simulink model "model"  (R2025a)
settings: Solver=ode4  StartTime=0.0  StopTime=350  FixedStep=fsw.sim.Ts  RelTol=1e-3
values from neighbouring files (symbols this model uses):
  const = load_constants()    [main.m]
  fsw = load_fsw(hw)    [main.m]
  hw = load_hardware()    [main.m]
  ic = load_ic(const, scn)    [main.m]
  scn = load_scenario(const)    [main.m]
  type = scn.type    [main.m]
undefined symbols (not defined in the file or in its folder): FK5, IAU
libraries: vrlib x13, aerolibutil x9, simulink x4, simulink_extras x3, slpidlib x1, aerolibtransform2 x1, aerolibatmos2 x1
settings Model: Creator=procyon  LastModifiedBy=procyon
settings SolverCC: MinimalZcImpactIntegration=on
settings DebuggingCC: ReadBeforeWriteMsg=DisableAll  WriteAfterWriteMsg=DisableAll  WriteAfterReadMsg=DisableAll  MultiTaskDSMMsg=none
settings ModelReferenceCC: UpdateModelReferenceTargets=IfOutOfDate
settings SFSimCC: SFSimEcho=off

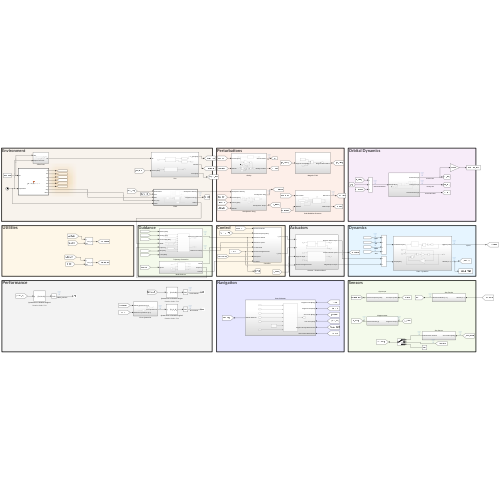
[thumbnail: Simulink's stored preview of the top-level diagram]
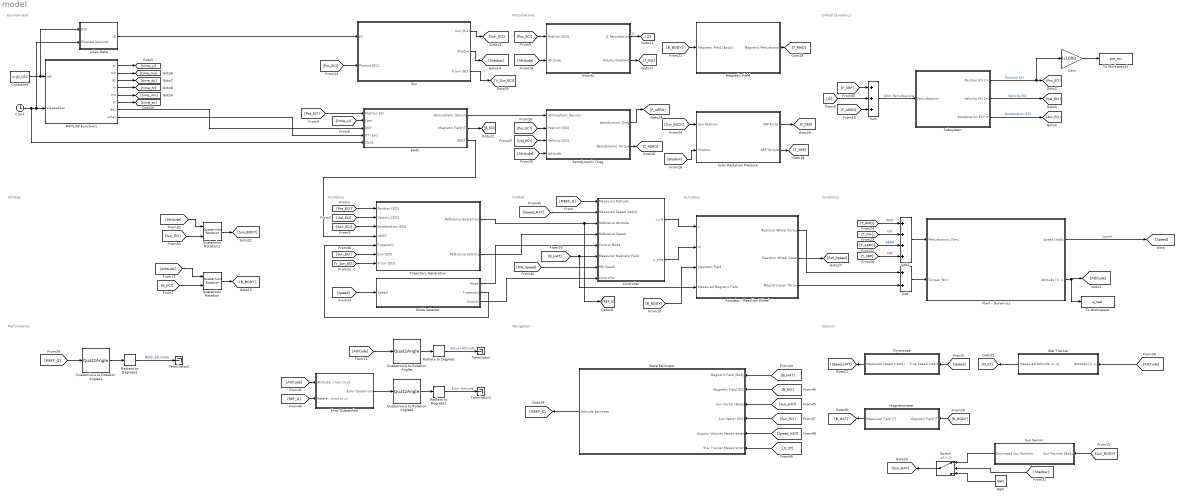
== system model ==
  note: Utilities
  note: Performance
  note: Guidance
  note: Orbital Dynamics
  note: Environment
  note: Navigation
  note: Sensors
  note: Perturbations
  note: Control
  note: Actuators
  note: Dynamics
  Actuator - Reaction Wheel : Subsystem
  Add : Sum
  Add1 : Sum  Inputs=++++
  Aerodynamic Drag : Subsystem
  Clock : Clock
  Constant4 : Constant  Value=ic.JD_UTC
  Controller : Subsystem
  Earth : Subsystem  TreatAsAtomicUnit=on  SystemSampleTime=fsw.sim.Tenv
  Error Quaternion : Subsystem
  Gain : Gain  Gain=1/1000
  Gravity : Subsystem
  Gyroscope : Subsystem
  Julian Date : Subsystem
  MATLAB Function1 : MATLAB Function  TreatAsAtomicUnit=on
  Magnetic Field : Subsystem
  Magnetometer : Subsystem
  Mode Selector : Subsystem
  NaN : Constant  Value=NaN  OutDataTypeStr=Inherit: Inherit via back propagation
  Plant - Dynamics : Subsystem
  Quaternion Rotation : aerolibutil/Quaternion Rotation
  Quaternion Rotation1 : aerolibutil/Quaternion Rotation
  Quaternions to Rotation Angles : Quat2Angle
      settings: AttributesFormatString=Rotation Order: %<rotationOrder>
  Quaternions to Rotation Angles1 : Quat2Angle
      settings: AttributesFormatString=Rotation Order: %<rotationOrder>
  Quaternions to Rotation Angles2 : Quat2Angle
      settings: AttributesFormatString=Rotation Order: %<rotationOrder>
  Radians to Degrees : simulink_extras/Transformations/Radians to Degrees
  Radians to Degrees1 : simulink_extras/Transformations/Radians to Degrees
  Radians to Degrees2 : simulink_extras/Transformations/Radians to Degrees
  Solar Radiation Pressure : Subsystem
  Star Tracker : Subsystem
  State Estimator : Subsystem
  Subsystem : Subsystem
  Sum : Sum  Inputs=+++
  Sun : Subsystem
  Sun Sensor : Subsystem
  Switch : Switch  Criteria=u2 > Threshold  SaturateOnIntegerOverflow=off  InputSameDT=off
  Terminator : Terminator
  Terminator1 : Terminator
  Terminator2 : Terminator
  To Workspace : ToWorkspace  VariableName=q_real  SaveFormat=Timeseries  SampleTime=-1
  To Workspace1 : ToWorkspace  VariableName=pos_eci  SaveFormat=Timeseries  SampleTime=-1
  Trajectory Generation : Subsystem
  wires:
  Plant - Dynamics/1(Speed [rad/s]) -> [Speed]  "Speed"
  Controller/1(u_rw) -> Actuator - Reaction Wheel/1(u)
  Plant - Dynamics/2(Attitude [n. u.]) -> [Attitude], To Workspace/1
  Subsystem/1(Position ECI [m]) -> Gain/1, [Pos_ECI]  "Position ECI"
  Subsystem/3(Acceleration ECI [m]) -> [Acc_ECI]  "Acceleration ECI"
  Subsystem/2(Velocity ECI [m]) -> [Vel_ECI]  "Velocity ECI"
  MATLAB Function1/1(yr) -> [time_yr]
  MATLAB Function1/2(mo) -> [time_mo]
  MATLAB Function1/3(dy) -> [time_dy]
  MATLAB Function1/4(hr) -> [time_hr]
  MATLAB Function1/5(mn) -> [time_mn]
  MATLAB Function1/6(sc) -> [time_sc]
  Constant4/1 -> Julian Date/1(JD0), MATLAB Function1/1(jd0)
  Clock/1 -> Earth/5(Clock), Julian Date/2(Elapsed Seconds), MATLAB Function1/2(elapsedSec)
  [Pos_ECI] -> Trajectory Generation/1(Position [ECI])
  [Vel_ECI] -> Trajectory Generation/2(Velocity [ECI])
  [Acc_ECI] -> Trajectory Generation/3(Acceleration [ECI])
  Trajectory Generation/1(Reference Quaternion) -> [REF_Q], Controller/3(Reference Attitude)
  Trajectory Generation/2(Reference Velocity) -> Controller/4(Reference Speed)
  Gain/1 -> To Workspace1/1
  [Pos_ECI] -> Earth/1(Position ECI)
  [Speed] -> Gyroscope/1(True Speed [rad/s])
  MATLAB Function1/7(doy) -> Earth/3(DOY)
  [time_yr] -> Earth/2(Year)
  MATLAB Function1/8(utSec) -> Earth/4(UT (sec))
  Gravity/1(J2 Perturbation) -> [J2]  "J2"
  [Pos_ECI] -> Gravity/1(Position [ECI])
  Controller/2(u_mtq) -> Actuator - Reaction Wheel/2(m)
  [B_BODY] -> Actuator - Reaction Wheel/3(Magnetic Field)
  Radians to Degrees/1 -> Terminator/1  "Actual Attitude"
  Quaternions to Rotation Angles/1 -> Radians to Degrees/1
  [Attitude] -> Quaternions to Rotation Angles/1
  Actuator - Reaction Wheel/1(Reaction Wheel Torque) -> Add/1
  Actuator - Reaction Wheel/3(Magnetorquer Torque) -> Add/2
  [Speed] -> Mode Selector/1(Speed)
  [Pos_ECI] -> Sun/2(Postion [ECI])
  Julian Date/1(JD) -> Sun/1(JD)
  Sun/1(Sun [ECI]) -> [Sun_ECI]
  Earth/1(Atmospheric Density) -> Aerodynamic Drag/1(Atmospheric Density)
  Sun/2(Shadow) -> [Shadow]
  [Sun_BODY] -> Solar Radiation Pressure/1(Sun Position)
  [Shadow] -> Solar Radiation Pressure/2(Shadow)
  [Attitude] -> Gravity/2(Attitude)
  Earth/3(GMST) -> Trajectory Generation/4(GMST)
  Earth/2(Magnetic Field [T]) -> [B_ECI]
  [B_ECI] -> Quaternion Rotation/2
  [Attitude] -> Quaternion Rotation/1
  Quaternion Rotation/1 -> [B_BODY]
  [B_BODY] -> Magnetic Field/1(Magnetic Field [Body])
  Add/1 -> Plant - Dynamics/2(Torque [Nm])
  Gravity/2(Gravity Gradient) -> [T_GG]
  Solar Radiation Pressure/2(SRP Torque) -> [T_SRP]
  Magnetic Field/1(Magnetic Perturbation) -> [T_RMD]
  [T_SRP] -> Add1/4  "SRP"
  [T_AERO] -> Add1/3  "AERO"
  [T_GG] -> Add1/2  "GG"
  [T_RMD] -> Add1/1  "RMD"
  [Attitude] -> Aerodynamic Drag/4(Attitude)
  [Pos_ECI] -> Aerodynamic Drag/2(Position [ECI])
  [Vel_ECI] -> Aerodynamic Drag/3(Velocity [ECI])
  Add1/1 -> Plant - Dynamics/1(Perturbations [Nm])
  [B_BODY] -> Magnetometer/1(Magnetic Field [T])
  Magnetometer/1(Measured Field [T]) -> [B_HAT]
  [B_HAT] -> Actuator - Reaction Wheel/4(Measured Magnetic Field), Controller/6(Measured Magnetic Field)
  Gyroscope/1(Measured Speed [rad/s]) -> [Speed_HAT]
  [Speed_HAT] -> Controller/2(Measured Speed [rad/s])
  [Shadow] -> Switch/2
  [Attitude] -> Quaternion Rotation1/1
  [Sun_ECI] -> Quaternion Rotation1/2
  Quaternion Rotation1/1 -> [Sun_BODY]
  [Sun_BODY] -> Sun Sensor/1(Sun Position [Body])
  [Attitude] -> Star Tracker/1(Attitude [n. u.])
  Star Tracker/1(Measured Attitude [n. u]) -> [Q_ST]
  Quaternions to Rotation Angles1/1 -> Radians to Degrees1/1
  Radians to Degrees1/1 -> Terminator2/1  "MEKF_Estimate"
  State Estimator/1(Attitude Estimate) -> [MEKF_Q]
  [B_HAT] -> State Estimator/1(Magnetic Field [Body])
  [B_ECI] -> State Estimator/2(Magnetic Field [ECI])
  [Sun_HAT] -> State Estimator/3(Sun Vector [Body])
  [Sun_ECI] -> State Estimator/4(Sun Vector [ECI])
  [Speed_HAT] -> State Estimator/5(Angular Velocity Measurement)
  [Q_ST] -> State Estimator/6(Star Tracker Measurement)
  [MEKF_Q] -> Quaternions to Rotation Angles1/1
  [MEKF_Q] -> Controller/1(Measured Attitude)
  Quaternions to Rotation Angles2/1 -> Radians to Degrees2/1
  Radians to Degrees2/1 -> Terminator1/1  "Error Attitude"
  [REF_Q] -> Error Quaternion/2(Reference Quaternion [n.u])
  [Attitude] -> Error Quaternion/1(Attitude Quaternion [n.u])
  Error Quaternion/1(Error Quaternion) -> Quaternions to Rotation Angles2/1
  Sun Sensor/1(Estimated Sun Position) -> Switch/1
  Switch/1 -> [Sun_HAT]
  NaN/1 -> Switch/3
  Actuator - Reaction Wheel/2(Reaction Wheel Speed) -> [RW_Speed]
  [RW_Speed] -> Controller/7(RW Speed)
  Aerodynamic Drag/2(Aerodynamic Torque) -> [T_AERO]
  Aerodynamic Drag/1(Aerodynamic Drag) -> [F_AERO]
  Solar Radiation Pressure/1(SRP Force) -> [F_SRP]
  Sum/1 -> Subsystem/1(Perturbations)  "Orbit Perturbations"
  [J2] -> Sum/2
  [F_SRP] -> Sum/1
  [F_AERO] -> Sum/3
  Mode Selector/2(Trajectory) -> Trajectory Generation/5(Trajectory)
  Mode Selector/1(Mode) -> Controller/5(Control Mode)
  Mode Selector/3(Control) -> Controller/8(Controller)
  Sun/3(V Sun [ECI]) -> [V_Sun_ECI]
  [V_Sun_ECI] -> Trajectory Generation/7(V Sun [ECI])
  [Sun_ECI] -> Trajectory Generation/6(Sun [ECI])

== system model/Actuator - Reaction Wheel ==
  u : Inport
  m : Inport  Port=2
  Magnetic Field : Inport  Port=3
  Measured Magnetic Field : Inport  Port=4
  DC Motor : Subsystem
  Magnetorquer : Subsystem
  PI Control : Subsystem
  Reaction Wheel Torque : Outport
  Reaction Wheel Speed : Outport  Port=2
  Magnetorquer Torque : Outport  Port=3
  wires:
  DC Motor/2(Speed [rad/s]) -> Reaction Wheel Speed/1, PI Control/2(Motor Speed)
  u/1 -> PI Control/1(Motor Reference)
  Magnetorquer/1(Torque [N.m]) -> Magnetorquer Torque/1
  Magnetic Field/1 -> Magnetorquer/2(Magnetic Field)
  m/1 -> Magnetorquer/1(u_mtq)
  DC Motor/1(Torque [N.m]) -> Reaction Wheel Torque/1
  Measured Magnetic Field/1 -> Magnetorquer/3(Measured Magnetic Field)
  PI Control/1(Voltage) -> DC Motor/1(Voltage)

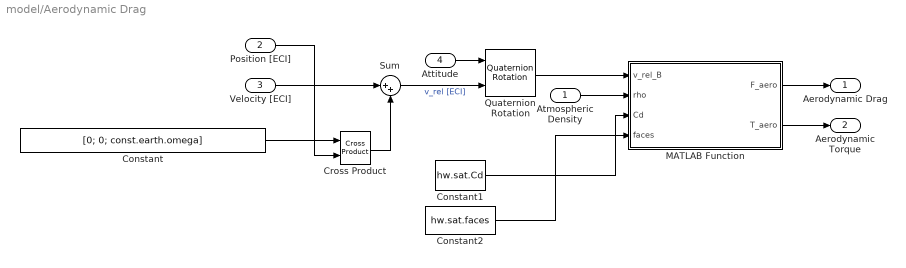
== system model/Aerodynamic Drag ==
  Atmospheric Density : Inport
  Position [ECI] : Inport  Port=2
  Velocity [ECI] : Inport  Port=3
  Attitude : Inport  Port=4
  Constant : Constant  Value=[0; 0; const.earth.omega]
  Constant1 : Constant  Value=hw.sat.Cd
  Constant2 : Constant  Value=hw.sat.faces
  Cross Product : vrlib/Utilities/Cross Product
  MATLAB Function : MATLAB Function  TreatAsAtomicUnit=on
  Quaternion Rotation : aerolibutil/Quaternion Rotation
  Sum : Sum  Inputs=|++
  Aerodynamic Drag : Outport
  Aerodynamic Torque : Outport  Port=2
  wires:
  Constant/1 -> Cross Product/1
  Position [ECI]/1 -> Cross Product/2
  Velocity [ECI]/1 -> Sum/1
  Cross Product/1 -> Sum/2
  Attitude/1 -> Quaternion Rotation/1
  Sum/1 -> Quaternion Rotation/2  "v_rel [ECI]"
  Quaternion Rotation/1 -> MATLAB Function/1(v_rel_B)
  Atmospheric Density/1 -> MATLAB Function/2(rho)
  Constant1/1 -> MATLAB Function/3(Cd)
  Constant2/1 -> MATLAB Function/4(faces)
  MATLAB Function/1(F_aero) -> Aerodynamic Drag/1
  MATLAB Function/2(T_aero) -> Aerodynamic Torque/1

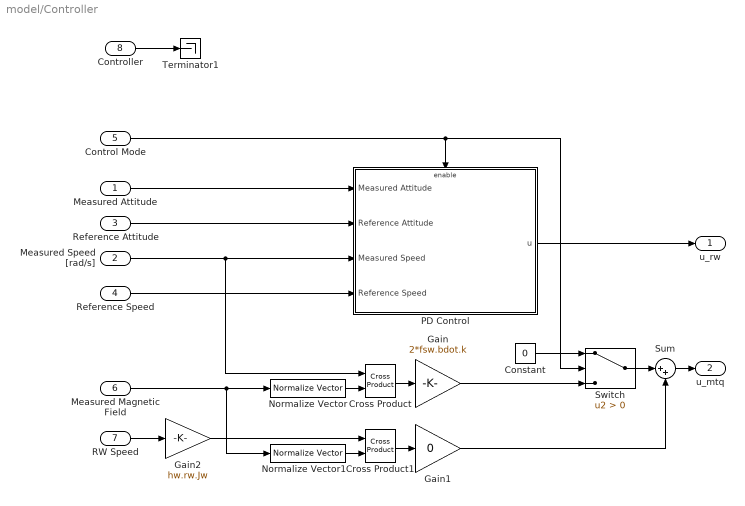
== system model/Controller ==
  Measured Attitude : Inport
  Measured Speed [rad/s] : Inport  Port=2
  Reference Attitude : Inport  Port=3
  Reference Speed : Inport  Port=4
  Control Mode : Inport  Port=5
  Measured Magnetic Field : Inport  Port=6
  RW Speed : Inport  Port=7
  Controller : Inport  Port=8
  Constant : Constant  Value=0
  Cross Product : vrlib/Utilities/Cross Product
  Cross Product1 : vrlib/Utilities/Cross Product
  Gain : Gain  Gain=2*fsw.bdot.k
  Gain1 : Gain  Gain=0
  Gain2 : Gain  Gain=hw.rw.Jw
  Normalize Vector : vrlib/Utilities/Normalize Vector  maxzero=0
  Normalize Vector1 : vrlib/Utilities/Normalize Vector  maxzero=0
  PD Control : Subsystem
  Sum : Sum  Inputs=|++
  Switch : Switch  Criteria=u2 > Threshold  SaturateOnIntegerOverflow=off  InputSameDT=off
  Terminator1 : Terminator
  u_rw : Outport
  u_mtq : Outport  Port=2
  wires:
  Normalize Vector/1 -> Cross Product/2
  Cross Product/1 -> Gain/1
  Measured Magnetic Field/1 -> Normalize Vector1/1, Normalize Vector/1
  RW Speed/1 -> Gain2/1
  Controller/1 -> Terminator1/1
  Measured Attitude/1 -> PD Control/1(Measured Attitude)
  Measured Speed [rad/s]/1 -> PD Control/3(Measured Speed), Cross Product/1
  Reference Attitude/1 -> PD Control/2(Reference Attitude)
  Reference Speed/1 -> PD Control/4(Reference Speed)
  Control Mode/1 -> Switch/2, PD Control/Enable
  Cross Product1/1 -> Gain1/1
  Normalize Vector1/1 -> Cross Product1/2
  Gain2/1 -> Cross Product1/1
  Gain/1 -> Switch/3
  Gain1/1 -> Sum/2
  Switch/1 -> Sum/1
  Sum/1 -> u_mtq/1
  PD Control/1(u) -> u_rw/1
  Constant/1 -> Switch/1

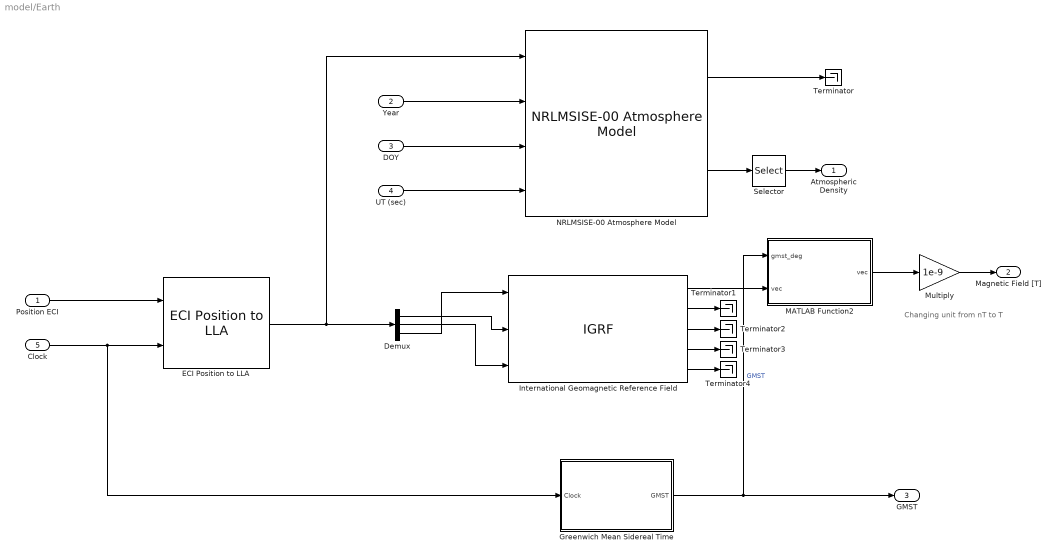
== system model/Earth ==
  note: Changing unit from nT to T
  Position ECI : Inport
  Year : Inport  Port=2
  DOY : Inport  Port=3
  UT (sec) : Inport  Port=4
  Clock : Inport  Port=5
  Demux : Demux  Outputs=3
  ECI Position to LLA : aerolibtransform2/ECI Position to LLA  red=IAU-76/FK5  year=2000  month=January  day=1  hour=12  min=0  sec=0  deltaT=Sec  errorflag=Error  extraparamflag=off  eunits=Metric (MKS)  earthmodel=WGS84  flat=1/298.257223563  eqradius=6378137
      settings: AttributesFormatString=%<red>
  Greenwich Mean Sidereal Time : Subsystem
  International Geomagnetic Reference Field : IGRF  time_in=off  month=January  day=1  year=2000  sv_out=off
      settings: AttributesFormatString=%<generation>
  MATLAB Function2 : MATLAB Function  TreatAsAtomicUnit=on
  Multiply : Gain  Gain=1e-9
  NRLMSISE-00 Atmosphere Model : aerolibatmos2/NRLMSISE-00 Atmosphere Model  units=Metric (MKS)  lst_input=off  flux_ap_input=off  flags_input=Internal  flags=ones(1,23)  oxygen_in=off  action=Warning
  Selector : Selector  InputPortWidth=9  IndexOptions=Index vector (dialog)  Indices=[6]  OutputSizes=1
  Terminator{,1..4} (5 alike) : Terminator
  Atmospheric Density : Outport
  Magnetic Field [T] : Outport  Port=2
  GMST : Outport  Port=3
  wires:
  ECI Position to LLA/1 -> Demux/1, NRLMSISE-00 Atmosphere Model/1
  NRLMSISE-00 Atmosphere Model/1 -> Terminator/1
  Position ECI/1 -> ECI Position to LLA/1
  Clock/1 -> Greenwich Mean Sidereal Time/1(Clock), ECI Position to LLA/2
  UT (sec)/1 -> NRLMSISE-00 Atmosphere Model/4
  DOY/1 -> NRLMSISE-00 Atmosphere Model/3
  Year/1 -> NRLMSISE-00 Atmosphere Model/2
  Demux/3 -> International Geomagnetic Reference Field/1
  Demux/1 -> International Geomagnetic Reference Field/2
  Demux/2 -> International Geomagnetic Reference Field/3
  International Geomagnetic Reference Field/2 -> Terminator1/1
  International Geomagnetic Reference Field/3 -> Terminator2/1
  International Geomagnetic Reference Field/4 -> Terminator3/1
  International Geomagnetic Reference Field/5 -> Terminator4/1
  NRLMSISE-00 Atmosphere Model/2 -> Selector/1
  Selector/1 -> Atmospheric Density/1
  MATLAB Function2/1(vec) -> Multiply/1
  Greenwich Mean Sidereal Time/1(GMST) -> MATLAB Function2/1(gmst_deg), GMST/1  "GMST"
  International Geomagnetic Reference Field/1 -> MATLAB Function2/2("vec ")
  Multiply/1 -> Magnetic Field [T]/1

== system model/Error Quaternion ==
  Attitude Quaternion [n.u] : Inport
  Reference Quaternion [n.u] : Inport  Port=2
  Quaternion Inverse : aerolibutil/Quaternion Inverse
  Quaternion Multiplication : aerolibutil/Quaternion Multiplication
  Error Quaternion : Outport
  wires:
  Reference Quaternion [n.u]/1 -> Quaternion Inverse/1
  Quaternion Multiplication/1 -> Error Quaternion/1
  Quaternion Inverse/1 -> Quaternion Multiplication/2
  Attitude Quaternion [n.u]/1 -> Quaternion Multiplication/1

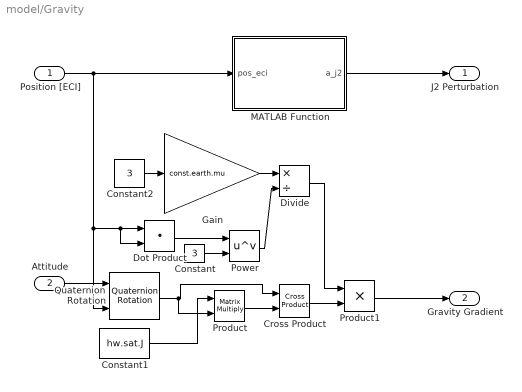
== system model/Gravity ==
  Position [ECI] : Inport
  Attitude : Inport  Port=2
  Constant : Constant  Value=3
  Constant1 : Constant  Value=hw.sat.J
  Constant2 : Constant  Value=3
  Cross Product : vrlib/Utilities/Cross Product
  Divide : Product  Inputs=*/
  Dot Product : DotProduct  OutDataTypeStr=Inherit: Inherit via internal rule
  Gain : Gain  Gain=const.earth.mu
  MATLAB Function : MATLAB Function  TreatAsAtomicUnit=on
  Power : Math  Operator=pow
  Product : Product  Multiplication=Matrix(*)
  Product1 : Product
  Quaternion Rotation : aerolibutil/Quaternion Rotation
  J2 Perturbation : Outport
  Gravity Gradient : Outport  Port=2
  wires:
  MATLAB Function/1(a_j2) -> J2 Perturbation/1
  Attitude/1 -> Quaternion Rotation/1
  Position [ECI]/1 -> MATLAB Function/1(pos_eci), Quaternion Rotation/2, Dot Product/2, Dot Product/1
  Power/1 -> Divide/2
  Dot Product/1 -> Power/1
  Constant/1 -> Power/2
  Quaternion Rotation/1 -> Product/2, Cross Product/1
  Constant1/1 -> Product/1
  Product/1 -> Cross Product/2
  Cross Product/1 -> Product1/2
  Constant2/1 -> Gain/1
  Gain/1 -> Divide/1
  Divide/1 -> Product1/1
  Product1/1 -> Gravity Gradient/1

== system model/Gyroscope ==
  True Speed [rad/s] : Inport
  Add : Sum  Inputs=+++
  Bias : simulink/Sources/Band-Limited White Noise  Cov=hw.gyro.sigma_bias^2  Ts=fsw.sim.Ts  seed=[23341]
  Integrator : Integrator  InitialCondition=hw.gyro.bias0
  Noise : simulink/Sources/Band-Limited White Noise  Cov=hw.gyro.sigma_noise^2  Ts=fsw.sim.Ts  seed=[23341]
  Measured Speed [rad/s] : Outport
  wires:
  True Speed [rad/s]/1 -> Add/2
  Add/1 -> Measured Speed [rad/s]/1
  Noise/1 -> Add/1
  Integrator/1 -> Add/3
  Bias/1 -> Integrator/1

== system model/Julian Date ==
  JD0 : Inport
  Elapsed Seconds : Inport  Port=2
  Constant : Constant  Value=86400
  Divide : Product  Inputs=*/
  Sum : Sum  Inputs=|++
  JD : Outport
  wires:
  Elapsed Seconds/1 -> Divide/1
  Constant/1 -> Divide/2
  JD0/1 -> Sum/1
  Sum/1 -> JD/1
  Divide/1 -> Sum/2

== system model/Magnetic Field ==
  Magnetic Field [Body] : Inport
  Constant : Constant  Value=hw.sat.rmd
  Cross Product : vrlib/Utilities/Cross Product
  Magnetic Perturbation : Outport
  wires:
  Cross Product/1 -> Magnetic Perturbation/1
  Magnetic Field [Body]/1 -> Cross Product/2
  Constant/1 -> Cross Product/1

== system model/Magnetometer ==
  Magnetic Field [T] : Inport
  Add : Sum  Inputs=+++
  Constant : Constant  Value=hw.mag.bias
  Noise : simulink/Sources/Band-Limited White Noise  Cov=hw.mag.sigma_noise^2 * hw.mag.dt  Ts=fsw.sim.Ts  seed=[23341]
  Zero-Order Hold : ZeroOrderHold  SampleTime=hw.mag.dt
  Measured Field [T] : Outport
  wires:
  Add/1 -> Zero-Order Hold/1
  Noise/1 -> Add/1
  Constant/1 -> Add/3
  Magnetic Field [T]/1 -> Add/2
  Zero-Order Hold/1 -> Measured Field [T]/1

== system model/Mode Selector ==
  Speed : Inport
  Clock : Clock
  Constant : Constant  Value=type
  MATLAB Function : MATLAB Function  TreatAsAtomicUnit=on
  Mode : Outport
  Trajectory : Outport  Port=2
  Control : Outport  Port=3
  wires:
  Speed/1 -> MATLAB Function/1(w)
  MATLAB Function/1(mode) -> Mode/1
  MATLAB Function/3(ctrl_select) -> Control/1
  MATLAB Function/2(traj_select) -> Trajectory/1
  Constant/1 -> MATLAB Function/2(scn_type)
  Clock/1 -> MATLAB Function/3(t)

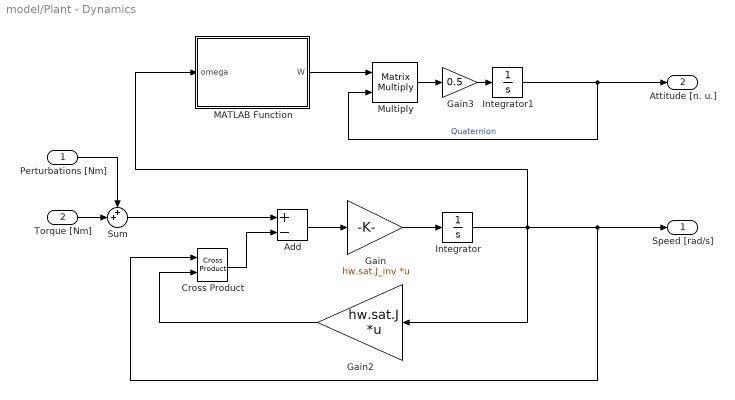
== system model/Plant - Dynamics ==
  Perturbations [Nm] : Inport
  Torque [Nm] : Inport  Port=2
  Add : Sum  Inputs=+-
  Cross Product : vrlib/Utilities/Cross Product
  Gain : Gain  Gain=hw.sat.J_inv  Multiplication=Matrix(K*u) (u vector)
  Gain2 : Gain  Gain=hw.sat.J  Multiplication=Matrix(K*u) (u vector)
  Gain3 : Gain  Gain=0.5
  Integrator : Integrator  InitialCondition=ic.w0
  Integrator1 : Integrator  InitialCondition=ic.q0
  MATLAB Function : MATLAB Function  TreatAsAtomicUnit=on
  Multiply : Product  Inputs=**  Multiplication=Matrix(*)
  Sum : Sum  Inputs=++|
  Speed [rad/s] : Outport
  Attitude [n. u.] : Outport  Port=2
  wires:
  Add/1 -> Gain/1
  Cross Product/1 -> Add/2
  Gain2/1 -> Cross Product/2
  Integrator/1 -> MATLAB Function/1(omega), Cross Product/1, Speed [rad/s]/1, Gain2/1
  MATLAB Function/1(W) -> Multiply/1
  Multiply/1 -> Gain3/1
  Integrator1/1 -> Attitude [n. u.]/1, Multiply/2  "Quaternion"
  Gain3/1 -> Integrator1/1
  Gain/1 -> Integrator/1
  Perturbations [Nm]/1 -> Sum/1
  Torque [Nm]/1 -> Sum/2
  Sum/1 -> Add/1

== system model/Solar Radiation Pressure ==
  Sun Position : Inport
  Shadow : Inport  Port=2
  Constant : Constant  Value=const.phys.c
  Constant1 : Constant  Value=const.sun.solar_const
  Constant2 : Constant  Value=hw.sat.faces
  MATLAB Function : MATLAB Function  TreatAsAtomicUnit=on
  SRP Force : Outport
  SRP Torque : Outport  Port=2
  wires:
  Constant/1 -> MATLAB Function/3(c)
  Constant1/1 -> MATLAB Function/2(solar_const)
  Constant2/1 -> MATLAB Function/4(faces)
  Sun Position/1 -> MATLAB Function/1(s_B)
  MATLAB Function/2(T_srp) -> SRP Torque/1
  MATLAB Function/1(F_srp) -> SRP Force/1

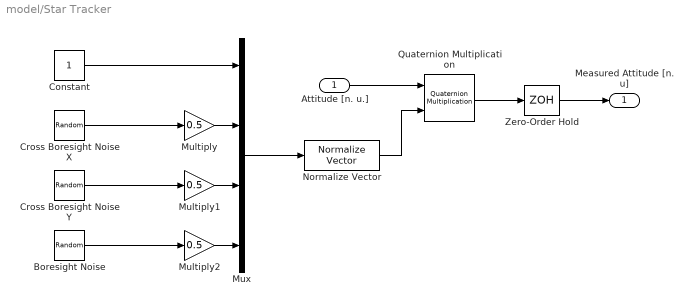
== system model/Star Tracker ==
  Attitude [n. u.] : Inport
  Boresight Noise : RandomNumber  Variance=hw.st.sigma_bore^2  SampleTime=hw.st.dt
  Constant : Constant
  Cross Boresight Noise X : RandomNumber  Variance=hw.st.sigma_cross^2  SampleTime=hw.st.dt
  Cross Boresight Noise Y : RandomNumber  Variance=hw.st.sigma_cross^2  SampleTime=hw.st.dt
  Multiply : Gain  Gain=0.5
  Multiply1 : Gain  Gain=0.5
  Multiply2 : Gain  Gain=0.5
  Mux : Mux
  Normalize Vector : vrlib/Utilities/Normalize Vector  maxzero=0
  Quaternion Multiplication : aerolibutil/Quaternion Multiplication
  Zero-Order Hold : ZeroOrderHold  SampleTime=0.1
  Measured Attitude [n. u] : Outport
  wires:
  Constant/1 -> Mux/1
  Cross Boresight Noise X/1 -> Multiply/1
  Cross Boresight Noise Y/1 -> Multiply1/1
  Boresight Noise/1 -> Multiply2/1
  Mux/1 -> Normalize Vector/1
  Attitude [n. u.]/1 -> Quaternion Multiplication/1
  Multiply/1 -> Mux/2
  Multiply1/1 -> Mux/3
  Multiply2/1 -> Mux/4
  Quaternion Multiplication/1 -> Zero-Order Hold/1
  Normalize Vector/1 -> Quaternion Multiplication/2
  Zero-Order Hold/1 -> Measured Attitude [n. u]/1

== system model/State Estimator ==
  Magnetic Field [Body] : Inport
  Magnetic Field [ECI] : Inport  Port=2
  Sun Vector [Body] : Inport  Port=3
  Sun Vector [ECI] : Inport  Port=4
  Angular Velocity Measurement : Inport  Port=5
  Star Tracker Measurement : Inport  Port=6
  Constant : Constant  Value=fsw.sim.Ts
  MATLAB Function : MATLAB Function  TreatAsAtomicUnit=on
  Attitude Estimate : Outport
  wires:
  Magnetic Field [Body]/1 -> MATLAB Function/1(mag_b)
  Magnetic Field [ECI]/1 -> MATLAB Function/2(mag_ref)
  Sun Vector [Body]/1 -> MATLAB Function/3(sun_b)
  Sun Vector [ECI]/1 -> MATLAB Function/4(sun_ref)
  Angular Velocity Measurement/1 -> MATLAB Function/5(gyro)
  Constant/1 -> MATLAB Function/6(dt)
  Star Tracker Measurement/1 -> MATLAB Function/7(q_st)
  MATLAB Function/1(q_est) -> Attitude Estimate/1

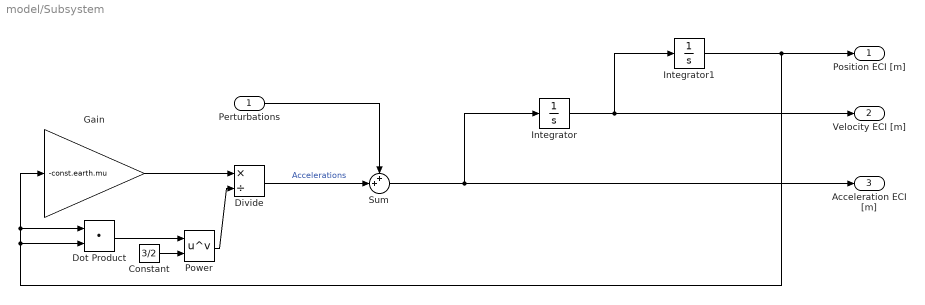
== system model/Subsystem ==
  Perturbations : Inport
  Constant : Constant  Value=3/2
  Divide : Product  Inputs=*/
  Dot Product : DotProduct  OutDataTypeStr=Inherit: Inherit via internal rule
  Gain : Gain  Gain=-const.earth.mu
  Integrator : Integrator  InitialCondition=ic.v0_I
  Integrator1 : Integrator  InitialCondition=ic.r0_I
  Power : Math  Operator=pow
  Sum : Sum  Inputs=++|
  Position ECI [m] : Outport
  Velocity ECI [m] : Outport  Port=2
  Acceleration ECI [m] : Outport  Port=3
  wires:
  Integrator/1 -> Integrator1/1, Velocity ECI [m]/1
  Integrator1/1 -> Dot Product/2, Dot Product/1, Gain/1, Position ECI [m]/1
  Dot Product/1 -> Power/1
  Gain/1 -> Divide/1
  Constant/1 -> Power/2
  Power/1 -> Divide/2
  Perturbations/1 -> Sum/1
  Divide/1 -> Sum/2  "Accelerations"
  Sum/1 -> Acceleration ECI [m]/1, Integrator/1

== system model/Sun ==
  JD : Inport
  Postion [ECI] : Inport  Port=2
  Eclipse Shadow Model (Cylindrical) : EclipseShadowModel  shadowModel=Cylindrical
  Normalize Vector : vrlib/Utilities/Normalize Vector  maxzero=0
  Normalize Vector1 : vrlib/Utilities/Normalize Vector  maxzero=0
  Planetary Ephemeris : PlanetaryEphem  target=Sun
  Sun [ECI] : Outport
  Shadow : Outport  Port=2
  V Sun [ECI] : Outport  Port=3
  wires:
  Planetary Ephemeris/1 -> Normalize Vector/1
  JD/1 -> Planetary Ephemeris/1
  Planetary Ephemeris/2 -> Normalize Vector1/1
  Postion [ECI]/1 -> Eclipse Shadow Model (Cylindrical)/1
  Eclipse Shadow Model (Cylindrical)/1 -> Shadow/1
  Normalize Vector/1 -> Sun [ECI]/1
  Normalize Vector1/1 -> V Sun [ECI]/1

== system model/Sun Sensor ==
  Sun Position [Body] : Inport
  Add : Sum
  Noise : simulink/Sources/Band-Limited White Noise  Cov=hw.ss.sigma_angle^2  Ts=fsw.sim.Ts  seed=[23341]
  Normalize Vector : vrlib/Utilities/Normalize Vector  maxzero=0
  Zero-Order Hold : ZeroOrderHold  SampleTime=hw.ss.dt
  Estimated Sun Position : Outport
  wires:
  Sun Position [Body]/1 -> Add/2
  Noise/1 -> Add/1
  Add/1 -> Normalize Vector/1
  Normalize Vector/1 -> Zero-Order Hold/1
  Zero-Order Hold/1 -> Estimated Sun Position/1

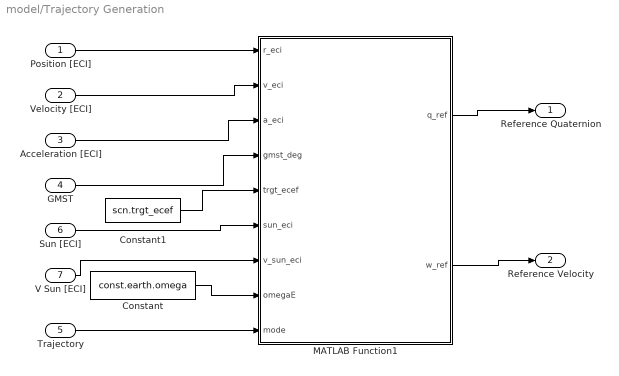
== system model/Trajectory Generation ==
  Position [ECI] : Inport
  Velocity [ECI] : Inport  Port=2
  Acceleration [ECI] : Inport  Port=3
  GMST : Inport  Port=4
  Trajectory : Inport  Port=5
  Sun [ECI] : Inport  Port=6
  V Sun [ECI] : Inport  Port=7
  Constant : Constant  Value=const.earth.omega
  Constant1 : Constant  Value=scn.trgt_ecef
  MATLAB Function1 : MATLAB Function  TreatAsAtomicUnit=on
  Reference Quaternion : Outport
  Reference Velocity : Outport  Port=2
  wires:
  Position [ECI]/1 -> MATLAB Function1/1(r_eci)
  Velocity [ECI]/1 -> MATLAB Function1/2(v_eci)
  Acceleration [ECI]/1 -> MATLAB Function1/3(a_eci)
  GMST/1 -> MATLAB Function1/4(gmst_deg)
  Constant1/1 -> MATLAB Function1/5(trgt_ecef)
  Constant/1 -> MATLAB Function1/8(omegaE)
  MATLAB Function1/1(q_ref) -> Reference Quaternion/1
  MATLAB Function1/2(w_ref) -> Reference Velocity/1
  Trajectory/1 -> MATLAB Function1/9(mode)
  Sun [ECI]/1 -> MATLAB Function1/6(sun_eci)
  V Sun [ECI]/1 -> MATLAB Function1/7(v_sun_eci)

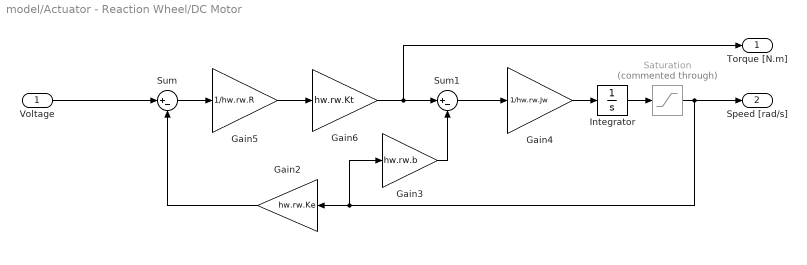
== system model/Actuator - Reaction Wheel/DC Motor ==
  Voltage : Inport
  Gain2 : Gain  Gain=hw.rw.Ke
  Gain3 : Gain  Gain=hw.rw.b
  Gain4 : Gain  Gain=1/hw.rw.Jw
  Gain5 : Gain  Gain=1/hw.rw.R
  Gain6 : Gain  Gain=hw.rw.Kt
  Integrator : Integrator
  Saturation : Saturate  Commented=through  UpperLimit=1000  LowerLimit=-1000
  Sum : Sum  Inputs=|+-
  Sum1 : Sum  Inputs=|+-
  Torque [N.m] : Outport
  Speed [rad/s] : Outport  Port=2
  wires:
  Voltage/1 -> Sum/1
  Gain2/1 -> Sum/2
  Sum/1 -> Gain5/1
  Gain6/1 -> Torque [N.m]/1, Sum1/1
  Integrator/1 -> Saturation/1
  Gain4/1 -> Integrator/1
  Gain5/1 -> Gain6/1
  Sum1/1 -> Gain4/1
  Gain3/1 -> Sum1/2
  Saturation/1 -> Gain3/1, Gain2/1, Speed [rad/s]/1

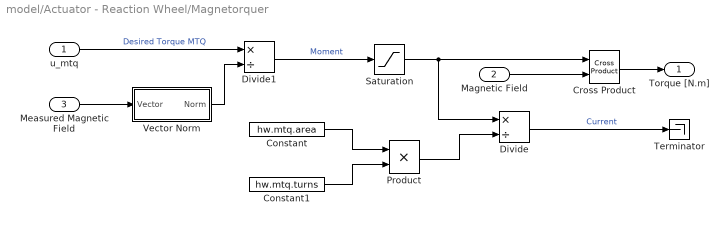
== system model/Actuator - Reaction Wheel/Magnetorquer ==
  u_mtq : Inport
  Magnetic Field : Inport  Port=2
  Measured Magnetic Field : Inport  Port=3
  Constant : Constant  Value=hw.mtq.area
  Constant1 : Constant  Value=hw.mtq.turns
  Cross Product : vrlib/Utilities/Cross Product
  Divide : Product  Inputs=*/
  Divide1 : Product  Inputs=*/
  Product : Product
  Saturation : Saturate  UpperLimit=hw.mtq.m_max  LowerLimit=-hw.mtq.m_max
  Terminator : Terminator
  Vector Norm : Subsystem
  Torque [N.m] : Outport
  wires:
  Magnetic Field/1 -> Cross Product/2
  Cross Product/1 -> Torque [N.m]/1
  Constant/1 -> Product/1
  Constant1/1 -> Product/2
  Product/1 -> Divide/2
  Divide/1 -> Terminator/1  "Current"
  Saturation/1 -> Cross Product/1, Divide/1
  Vector Norm/1(Norm) -> Divide1/2
  Measured Magnetic Field/1 -> Vector Norm/1(Vector)
  u_mtq/1 -> Divide1/1  "Desired Torque MTQ"
  Divide1/1 -> Saturation/1  "Moment"

== system model/Actuator - Reaction Wheel/PI Control ==
  Motor Reference : Inport
  Motor Speed : Inport  Port=2
  Gain : Gain  Gain=1/hw.rw.Jw
  Integrator : Integrator
  PID Controller : slpidlib/PID Controller  Controller=PI  Form=Parallel  TimeDomain=Continuous-time  UseExternalTs=off  SampleTime=-1  IntegratorMethod=Forward Euler  FilterMethod=Forward Euler  ControllerParametersSource=internal  P=0.3  I=2.3  UseKiTs=off  D=0  UseExternalDerivativeSource=off  N=100  UseFilter=on  TunerSelectOption=Transfer Function Based (PID Tuner App)  InitialConditionSource=internal  InitialConditionForIntegrator=0  InitialConditionForFilter=0  DifferentiatorICPrevScaledInput=0  ExternalReset=none  TrackingMode=off  Kt=1  LimitOutput=off  SatLimitsSource=internal  UpperSaturationLimit=inf  LowerSaturationLimit=-inf  LinearizeAsGain=on  AntiWindupMode=none  Kb=1  LimitIntegrator=off  UpperIntegratorSaturationLimit=inf  LowerIntegratorSaturationLimit=-inf  POutMin=[]  POutMax=[]  IOutMin=[]  IOutMax=[]  DOutMin=[]  DOutMax=[]  NOutMin=[]  NOutMax=[]  SumOutMin=[]  SumOutMax=[]  SaturationOutMin=[]  SaturationOutMax=[]  PParamMin=[]  PParamMax=[]  IParamMin=[]  IParamMax=[]  DParamMin=[]  DParamMax=[]  NParamMin=[]  NParamMax=[]  KbParamMin=[]  KbParamMax=[]  KtParamMin=[]  KtParamMax=[]  KbOutMin=[]  KbOutMax=[]  KtOutMin=[]  KtOutMax=[]  IntegratorOutMin=[]  IntegratorOutMax=[]  FilterOutMin=[]  FilterOutMax=[]  SumI1OutMin=[]  SumI1OutMax=[]  SumI2OutMin=[]  SumI2OutMax=[]  SumI3OutMin=[]  SumI3OutMax=[]  SumI4OutMin=[]  SumI4OutMax=[]  SumDOutMin=[]  SumDOutMax=[]  DifferentiatorOutMin=[]  DifferentiatorOutMax=[]  FilterDiffOutCoefMin=[]  FilterDiffOutCoefMax=[]  ReciprocalOutMin=[]  ReciprocalOutMax=[]  SumDenOutMin=[]  SumDenOutMax=[]  SumNumOutMin=[]  SumNumOutMax=[]  DivideOutMin=[]  DivideOutMax=[]  UdiffTsProdOutMin=[]  UdiffTsProdOutMax=[]  NTsProdOutMin=[]  NTsProdOutMax=[]  UintegralTsProdOutMin=[]  UintegralTsProdOutMax=[]  UngainTsProdOutMin=[]  UngainTsProdOutMax=[]  ClampingZeroOutDataTypeStr=Inherit: Inherit via back propagation  ClampingZeroOutMin=[]  ClampingZeroOutMax=[]  FilterDenConstantOutDataTypeStr=Inherit: Inherit via back propagation  FilterDenConstantOutMin=[]  FilterDenConstantOutMax=[]  PCopyOutDataTypeStr=Inherit: Inherit via back propagation  PCopyOutMin=[]  PCopyOutMax=[]  NCopyOutDataTypeStr=Inherit: Inherit via back propagation  NCopyOutMin=[]  NCopyOutMax=[]  IntegratorContinuousStateAttributes=''  IntegratorStateMustResolveToSignalObject=off  IntegratorRTWStateStorageClass=Auto  FilterContinuousStateAttributes=''  FilterStateMustResolveToSignalObject=off  FilterRTWStateStorageClass=Auto  ParallelPVariant=InternalParameters  IdealPVariant=Disabled  IVariant=InternalParameters  DVariant=Disabled  IntegratorVariant=Continuous  SatVariant=Disabled  AWVariant=Passthrough  PCopyVariant=Disabled  TRVariant=Disabled  FdbkBlocksVariant=Forward  IdealPFdbkVariant=Disabled  SatFdbkVariant=Disabled  DerivativeFilterVariant=Disabled  NVariant=Disabled  NCopyVariant=Disabled_SignalSpec  FilterICVariant=Disabled  IntegratorICVariant=InternalICs  ExternalResetVariant=Disabled  TRSumVariant=Passthrough  SumFdbkVariant=Disabled  SumVariant=Sum_PI  TsampFilterVariant=InternalTs  TsampNgainVariant=Passthrough  TsampIntegralVariant=Disabled_SignalSpec  ExternalSaturationOutDataTypeStr=Inherit: Same as second input  DerivativeSourceVariant=Disabled  PreIntVariant=InternalPreInt
  Sum : Sum  Inputs=|+-
  Voltage : Outport
  wires:
  Motor Reference/1 -> Gain/1
  Gain/1 -> Integrator/1
  Integrator/1 -> Sum/1
  Motor Speed/1 -> Sum/2
  Sum/1 -> PID Controller/1
  PID Controller/1 -> Voltage/1

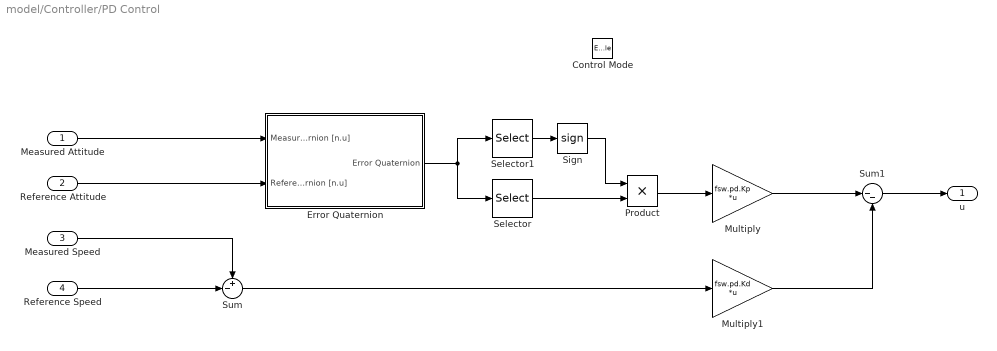
== system model/Controller/PD Control ==
  Measured Attitude : Inport
  Reference Attitude : Inport  Port=2
  Measured Speed : Inport  Port=3
  Reference Speed : Inport  Port=4
  Control Mode : EnablePort
  Error Quaternion : Subsystem
  Multiply : Gain  Gain=fsw.pd.Kp  Multiplication=Matrix(K*u) (u vector)
  Multiply1 : Gain  Gain=fsw.pd.Kd  Multiplication=Matrix(K*u) (u vector)
  Product : Product
  Selector : Selector  InputPortWidth=4  IndexOptions=Index vector (dialog)  Indices=[2 3 4]  OutputSizes=1
  Selector1 : Selector  InputPortWidth=4  IndexOptions=Index vector (dialog)  Indices=[1]  OutputSizes=1
  Sign : Signum
  Sum : Sum  Inputs=+-|
  Sum1 : Sum  Inputs=|--
  u : Outport
  wires:
  Error Quaternion/1(Error Quaternion) -> Selector1/1, Selector/1
  Selector1/1 -> Sign/1
  Selector/1 -> Product/2
  Product/1 -> Multiply/1
  Multiply/1 -> Sum1/1
  Sum/1 -> Multiply1/1
  Sign/1 -> Product/1
  Measured Attitude/1 -> Error Quaternion/1(Measured Quaternion [n.u])
  Reference Attitude/1 -> Error Quaternion/2(Reference Quaternion [n.u])
  Measured Speed/1 -> Sum/1
  Reference Speed/1 -> Sum/2
  Multiply1/1 -> Sum1/2
  Sum1/1 -> u/1

== system model/Earth/Greenwich Mean Sidereal Time ==
  Clock : Inport
  Add : Sum
  Constant : Constant  Value=ic.gmst0_deg
  Constant1 : Constant  Value=const.earth.omega
  Constant2 : Constant  Value=360
  Gain : Gain  Gain=180 / pi
  Mod : Math  Operator=mod
  Product : Product
  GMST : Outport
  wires:
  Clock/1 -> Product/2
  Constant1/1 -> Product/1
  Product/1 -> Gain/1
  Gain/1 -> Add/2
  Constant/1 -> Add/1
  Mod/1 -> GMST/1
  Add/1 -> Mod/1
  Constant2/1 -> Mod/2

== system model/Actuator - Reaction Wheel/Magnetorquer/Vector Norm ==
  Vector : Inport
  Dot Product : DotProduct  OutDataTypeStr=Inherit: Inherit via internal rule
  Square Root : Sqrt
  Norm : Outport
  wires:
  Vector/1 -> Dot Product/2, Dot Product/1
  Dot Product/1 -> Square Root/1
  Square Root/1 -> Norm/1

== system model/Controller/PD Control/Error Quaternion ==
  Measured Quaternion [n.u] : Inport
  Reference Quaternion [n.u] : Inport  Port=2
  Quaternion Inverse : aerolibutil/Quaternion Inverse
  Quaternion Multiplication : aerolibutil/Quaternion Multiplication
  Error Quaternion : Outport
  wires:
  Reference Quaternion [n.u]/1 -> Quaternion Inverse/1
  Quaternion Multiplication/1 -> Error Quaternion/1
  Quaternion Inverse/1 -> Quaternion Multiplication/2
  Measured Quaternion [n.u]/1 -> Quaternion Multiplication/1

== matlab function model/Trajectory Generation/MATLAB Function1 ==
  data: r_eci input; q_ref output; v_eci input; a_eci input; gmst_deg input; trgt_ecef input; sun_eci input; v_sun_eci input; omegaE input; mode input; w_ref output
%#codegen
function [q_ref, w_ref] = trajectory(r_eci, v_eci, a_eci, gmst_deg, trgt_ecef, sun_eci, v_sun_eci, omegaE, mode)

    q_ref = zeros(4,1);
    w_ref = zeros(3,1);

    r_eci = r_eci(:);
    v_eci = v_eci(:);
    a_eci = a_eci(:);
    sun_eci = sun_eci(:);
    v_sun_eci = v_sun_eci(:);

    switch mode
        case 1 % Inertial Pointing mode, satellite goes to origin
            q_ref = [1; 0; 0; 0];
            w_ref = [0; 0; 0];
        case 2 % Nadir Pointing mode, satellite points to Earth
            [q_ref, w_ref] = nadir_pointing(r_eci, v_eci, a_eci);
        case 3 % Sun Pointing mode, satellite points to the Sun
            [q_ref, w_ref] = sun_pointing(sun_eci, v_sun_eci, r_eci, v_eci, a_eci);
        case 4 % Target Tracking mode, satellite points to ground station
            [q_ref, w_ref] = target_tracking(gmst_deg, trgt_ecef, r_eci, v_eci, omegaE);
        otherwise
            q_ref = [1; 0; 0; 0];
            w_ref = [0; 0; 0];
    end

== matlab function model/Aerodynamic Drag/MATLAB Function ==
  data: F_aero output; v_rel_B input; T_aero output; rho input; Cd input; faces input
function [F_aero, T_aero] = aero_drag(v_rel_B, rho, Cd, faces)

    V = norm(v_rel_B);
    if V < eps
        F_aero = zeros(3,1);
        T_aero = zeros(3,1);
        return;
    end

    F_aero = zeros(3,1);
    T_aero = zeros(3,1);
    N = size(faces, 1);

    for k = 1:N
        n_k   = faces(k, 1:3)';
        A_k   = faces(k, 4);
        r_k   = faces(k, 5:7)';

        cos_alpha = dot(v_rel_B, n_k) / V;

        if cos_alpha > 0
            F_k = -0.5 * rho * Cd * A_k * cos_alpha * V * v_rel_B;
            F_aero = F_aero + F_k;
            T_aero = T_aero + cross(r_k, F_k);
        end
    end

end

== matlab function model/Plant - Dynamics/MATLAB Function ==
  data: omega input; W output
function W = omegaMat(omega)
%OMEGAMAT  Quaternion kinematic matrix (scalar-first convention)
%
%   Using the definition:
%       W(ω) = [  0      -ωᵀ
%                 ω   [ω×] ]

    % ensure column vector
    omega = omega(:);

    % skew-symmetric cross-product matrix
    omega_cross = [  0       -omega(3)   omega(2);
                  omega(3)     0        -omega(1);
                 -omega(2)   omega(1)     0      ];

    % assemble full 4x4 matrix
    W = [ 0          -omega.';
          omega       omega_cross ];
end

== matlab function model/MATLAB Function1 ==
  data: jd0 input; yr output; elapsedSec input; mo output; dy output; hr output; mn output; sc output; doy output; utSec output
function [yr, mo, dy, hr, mn, sc, doy, utSec] = julianToCalendar(jd0, elapsedSec)
%#codegen
% Converts initial Julian Date + elapsed seconds to calendar date/time.
%
% Inputs:
%   jd0        - Initial epoch as Julian Date (days)
%   elapsedSec - Elapsed simulation time (seconds)
%
% Outputs:
%   yr, mo, dy, hr, mn, sc - Current UTC date and time

    % Current Julian Date
    jd = jd0 + elapsedSec / 86400;

    % Algorithm based on Meeus, "Astronomical Algorithms"
    jd_plus = jd + 0.5;
    Z = floor(jd_plus);
    F = jd_plus - Z;

    if Z < 2299161
        A = Z;
    else
        alpha = floor((Z - 1867216.25) / 36524.25);
        A = Z + 1 + alpha - floor(alpha / 4);
    end

    B = A + 1524;
    C = floor((B - 122.1) / 365.25);
    D = floor(365.25 * C);
    E = floor((B - D) / 30.6001);

    day_frac = B - D - floor(30.6001 * E) + F;
    dy = floor(day_frac);

    if E < 14
        mo = E - 1;
    else
        mo = E - 13;
    end

    if mo > 2
        yr = C - 4716;
    else
        yr = C - 4715;
    end

    % Extract h/m/s from fractional day
    frac = day_frac - dy;
    hr = floor(frac * 24);
    mn = floor((frac * 24 - hr) * 60);
    sc = (frac * 86400) - hr * 3600 - mn * 60;

    % Extract DOY and UT (sec)
    daysInMonth = [31 28 31 30 31 30 31 31 30 31 30 31];
    if (mod(yr,4)==0 && mod(yr,100)~=0) || mod(yr,400)==0
        daysInMonth(2) = 29;
    end
    doy = sum(daysInMonth(1:mo-1)) + dy;

    utSec = hr * 3600 + mn * 60 + sc;
end

== matlab function model/Gravity/MATLAB Function ==
  data: pos_eci input; a_j2 output
function a_j2 = j2_perturbation(pos_eci)
    mu = 3.986004418e14;       % m^3/s^2
    R_E = 6378137;             % m
    J2 = 1.08263e-3;

    x = pos_eci(1);
    y = pos_eci(2);
    z = pos_eci(3);
    r = norm(pos_eci);

    k = -1.5 * J2 * mu * (R_E / r)^2 / r^2;

    a_j2 = k * [ (x/r) * (1 - 5*(z/r)^2);
                  (y/r) * (1 - 5*(z/r)^2);
                  (z/r) * (3 - 5*(z/r)^2) ];
end

== matlab function model/Mode Selector/MATLAB Function ==
  settings: updateMethod=DISCRETE  sampleTime=fsw.sim.Ts
  data: w input; scn_type input; mode output; traj_select output; ctrl_select output; t input
function [mode, traj_select, ctrl_select] = mission_mode(w, scn_type, t)
% MISSION_MODE  Finite-state mode selector with hysteresis and dwell timer.
%
%   [mode, traj_select, ctrl_select] = mission_mode(w, scn_type, t)
%
%   Selects between detumbling and pointing based on angular rate magnitude,
%   with a hysteresis band to prevent chatter near the threshold and a
%   minimum dwell time in pointing to ride out PD transients.
%
%   Inputs:
%       w        [3x1]  Angular velocity in body frame [rad/s]
%       scn_type [3x1]  Scenario configuration vector:
%                        (1) Scenario: 1 = single controller test (skip detumble)
%                                      2 = detumble + pointing
%                        (2) Pointing mode: 1 = inertial, 2 = nadir, 3 = sun, 4 = target
%                        (3) Controller:    1 = PD, 2 = LQR, 3 = SMC
%       t        Scalar Simulation time [s]
%
%   Outputs:
%       mode        Scalar  0 = detumble, 1 = pointing
%       traj_select Scalar  Trajectory generator selector (0 = none, else scn_type(2))
%       ctrl_select Scalar  Controller selector (0 = B-dot, else scn_type(3))

    %% Rate thresholds [rad/s]

    w_low  = 2.0 * pi/180;     % enter pointing below this
    w_high = 300.0 * pi/180;    % return to detumble above this

    %% Dwell time [s]

    t_dwell = 30;               % minimum time in pointing before allowing switch back

    %% Persistent state

    persistent state t_switch

    if isempty(state)
        if scn_type(1) == 1
            state = 1;          % test mode: start in pointing, never detumble
            t_switch = -inf;
        else
            state = 0;          % nominal: start in detumble
            t_switch = -inf;
        end
    end

    %% Hysteresis FSM (only active in scenario 2)

    if scn_type(1) == 2
        w_norm = norm(w);

        if state == 0 && w_norm < w_low
            state = 1;
            t_switch = t;       % latch transition time
        elseif state == 1 && w_norm > w_high && (t - t_switch) > t_dwell
            state = 0;
        end
    end

    %% Output mapping

    if state == 0
        mode        = 0;
        traj_select = 0;
        ctrl_select = 0;
    else
        mode        = 1;
        traj_select = scn_type(2);
        ctrl_select = scn_type(3);
    end

end

== matlab function model/Earth/MATLAB Function2 ==
  data: gmst_deg input; vec output; vec input
function vec = ecef2eci(gmst_deg, vec)

vec = vec(:); % Force column vector

% -------- ECI -> ECEF (from GMST) --------
th = gmst_deg * (pi/180);
c  = cos(th);
s  = sin(th);

C_ECI_ECEF = [ c -s 0;
               s  c 0;
               0  0 1];

vec = C_ECI_ECEF * vec; % Frame change from ECEF to ECI

== matlab function model/Solar Radiation Pressure/MATLAB Function ==
  data: F_srp output; s_B input; T_srp output; solar_const input; c input; faces input
function [F_srp, T_srp] = srp_torque(s_B, solar_const, c, faces)
% SRP_TORQUE  Solar radiation pressure torque in body frame.
%
%   T_srp = srp_torque(s_B, solar_const, c, faces)
%
%   Inputs:
%       s_B         - [3x1] unit vector from spacecraft to Sun (body frame)
%       solar_const - [1x1] solar constant [W/m^2]
%       c           - [1x1] speed of light [m/s]
%       faces       - [Nx10] each row: [nx ny nz  A  rx ry rz  cs cd ca]
%
%   Output:
%       T_srp       - [3x1] SRP torque about CoM [N·m]

    P = solar_const / c;       % radiation pressure [N/m^2]

    F_srp = zeros(3,1);
    T_srp = zeros(3,1);
    N = size(faces, 1);

    for k = 1:N
        n_k  = faces(k, 1:3)';
        A_k  = faces(k, 4);
        r_k  = faces(k, 5:7)';
        cs_k = faces(k, 8);
        cd_k = faces(k, 9);
        % ca_k = faces(k, 10);    % implicit: ca = 1 - cs - cd

        cos_theta = dot(s_B, n_k);

        if cos_theta > 0
            F_k = -P * A_k * cos_theta * ...
                  ((1 - cs_k) * s_B + 2 * (cs_k * cos_theta + cd_k / 3) * n_k);
            F_srp = F_srp + F_k;
            T_srp = T_srp + cross(r_k, F_k);
        end
    end

end

== matlab function model/State Estimator/MATLAB Function ==
  settings: updateMethod=DISCRETE  sampleTime=fsw.sim.Ts
  data: mag_b input; q_est output; mag_ref input; sun_b input; sun_ref input; gyro input; dt input; q_st input; mekf_cfg parameter
%#codegen
function q_est = mekf_compute(mag_b, mag_ref, sun_b, sun_ref, gyro, dt, q_st, mekf_cfg)
% MEKF_COMPUTE  Simulink interface wrapper for the MEKF.
%
%   Validates sensor inputs, determines measurement availability,
%   and calls mekf() with validity flags and configuration struct.
 
    % Enforce column vectors
    mag_b   = mag_b(:);    mag_ref = mag_ref(:);
    sun_b   = sun_b(:);    sun_ref = sun_ref(:);
    gyro    = gyro(:);
    q_st    = q_st(:);
 
    % Sensor validity
    mag_valid  = all(isfinite(mag_b))  && all(isfinite(mag_ref));
    sun_valid  = all(isfinite(sun_b))  && all(isfinite(sun_ref));
    gyro_valid = all(isfinite(gyro));
    st_valid   = all(isfinite(q_st));
 
    q_est = mekf(mag_b, mag_ref, sun_b, sun_ref, gyro, dt, q_st, ...
                 mag_valid, sun_valid, gyro_valid, st_valid, mekf_cfg);
end
